simulink model "quantization_distortion_power"  (R2016b)
settings: Solver=VariableStepAuto  StartTime=0.0  StopTime=100  MaxStep=0.001  RelTol=1e-3
settings Model: Creator=fhs42090  LastModifiedBy=fhs42090

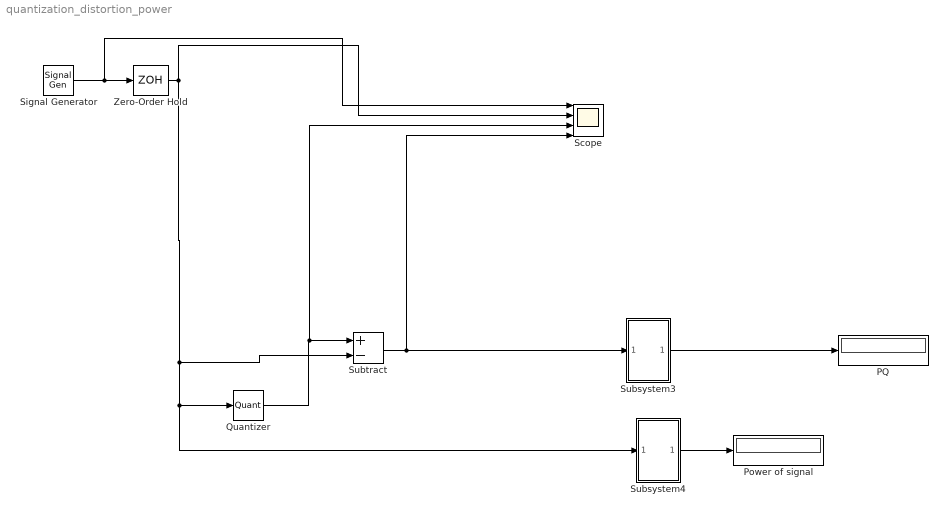
== system quantization_distortion_power ==
  PQ : Display
  Power of signal : Display
  Quantizer : Quantizer  QuantizationInterval=2/16
  Scope : Scope  NumInputPorts=4
  Signal Generator : SignalGenerator  Amplitude=1/10
  Subsystem3 : Subsystem
  Subsystem4 : Subsystem
  Subtract : Sum  Inputs=+-
  Zero-Order Hold : ZeroOrderHold  SampleTime=1/100
  wires:
  Zero-Order Hold/1 -> Scope/2, Subtract/2, Subsystem4/1(In1), Quantizer/1
  Signal Generator/1 -> Scope/1, Zero-Order Hold/1
  Quantizer/1 -> Scope/3, Subtract/1
  Subtract/1 -> Subsystem3/1(In1), Scope/4
  Subsystem3/1(Out1) -> PQ/1
  Subsystem4/1(Out1) -> Power of signal/1

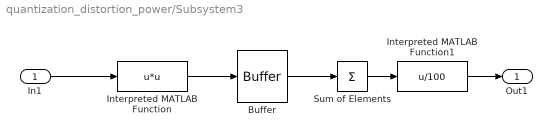
== system quantization_distortion_power/Subsystem3 ==
  In1 : Inport
  Buffer : Buffer  N=100  V=99  TreatMby1Signals=One channel  OutputFrames=off
  Interpreted MATLAB Function : MATLABFcn  MATLABFcn=u*u
  Interpreted MATLAB Function1 : MATLABFcn  MATLABFcn=u/100
  Sum of Elements : Sum  Inputs=+
  Out1 : Outport
  wires:
  In1/1 -> Interpreted MATLAB Function/1
  Interpreted MATLAB Function1/1 -> Out1/1
  Sum of Elements/1 -> Interpreted MATLAB Function1/1
  Buffer/1 -> Sum of Elements/1
  Interpreted MATLAB Function/1 -> Buffer/1

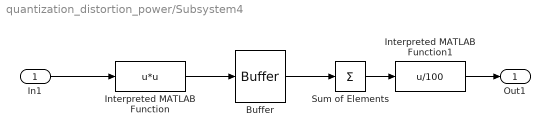
== system quantization_distortion_power/Subsystem4 ==
  In1 : Inport
  Buffer : Buffer  N=100  V=99  TreatMby1Signals=One channel  OutputFrames=off
  Interpreted MATLAB Function : MATLABFcn  MATLABFcn=u*u
  Interpreted MATLAB Function1 : MATLABFcn  MATLABFcn=u/100
  Sum of Elements : Sum  Inputs=+
  Out1 : Outport
  wires:
  Interpreted MATLAB Function/1 -> Buffer/1
  Buffer/1 -> Sum of Elements/1
  Sum of Elements/1 -> Interpreted MATLAB Function1/1
  Interpreted MATLAB Function1/1 -> Out1/1
  In1/1 -> Interpreted MATLAB Function/1
